simulink model "task2"  (R2024a)
settings: Solver=VariableStepAuto  StartTime=0.0  StopTime=10.0  MaxStep=0.01  RelTol=1e-3
undefined symbols (not defined in the file): Ab, Bb, Cb, D, Kb, L, xf0, xf0_hat
settings Model: Creator=sizgr  LastModifiedBy=sizgr

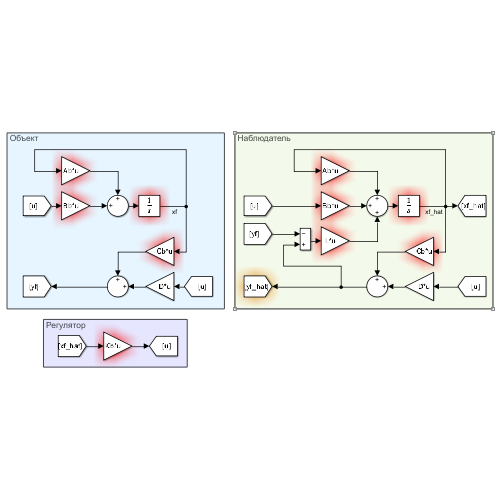
[thumbnail: Simulink's stored preview of the top-level diagram]
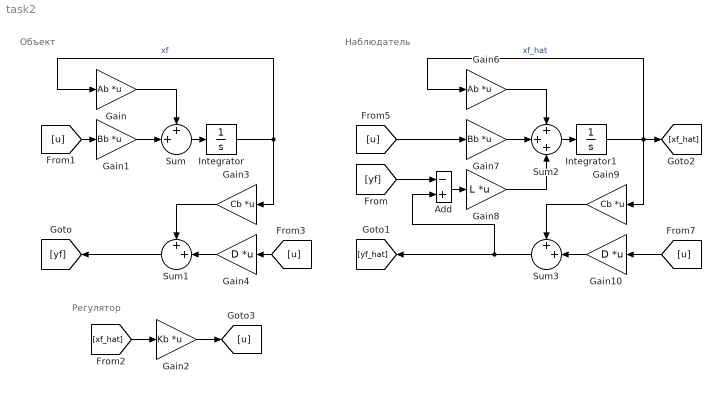
== system task2 ==
  note: Регулятор
  note: Объект
  note: Наблюдатель
  Add : Sum  Inputs=-+
  Gain : Gain  Gain=Ab  Multiplication=Matrix(K*u)
  Gain1 : Gain  Gain=Bb  Multiplication=Matrix(K*u)
  Gain10 : Gain  Gain=D  Multiplication=Matrix(K*u)
  Gain2 : Gain  Gain=Kb  Multiplication=Matrix(K*u)
  Gain3 : Gain  Gain=Cb  Multiplication=Matrix(K*u)
  Gain4 : Gain  Gain=D  Multiplication=Matrix(K*u)
  Gain6 : Gain  Gain=Ab  Multiplication=Matrix(K*u)
  Gain7 : Gain  Gain=Bb  Multiplication=Matrix(K*u)
  Gain8 : Gain  Gain=L  Multiplication=Matrix(K*u)
  Gain9 : Gain  Gain=Cb  Multiplication=Matrix(K*u)
  Integrator : Integrator  InitialCondition=xf0
  Integrator1 : Integrator  InitialCondition=xf0_hat
  Sum : Sum  Inputs=++|
  Sum1 : Sum  Inputs=++|
  Sum2 : Sum  Inputs=+++
  Sum3 : Sum  Inputs=++|
  wires:
  Sum/1 -> Integrator/1
  Integrator/1 -> Gain/1, Gain3/1  "xf"
  [u] -> Gain1/1
  Gain/1 -> Sum/1
  Gain1/1 -> Sum/2
  Gain4/1 -> Sum1/2
  [u] -> Gain4/1
  Gain3/1 -> Sum1/1
  Sum1/1 -> [yf]
  Gain9/1 -> Sum3/1
  [u] -> Gain10/1
  Gain10/1 -> Sum3/2
  Sum2/1 -> Integrator1/1
  Integrator1/1 -> Gain9/1, [xf_hat], Gain6/1  "xf_hat"
  Gain7/1 -> Sum2/2
  Sum3/1 -> Add/2, [yf_hat]
  Gain8/1 -> Sum2/3
  Add/1 -> Gain8/1
  [u] -> Gain7/1
  Gain6/1 -> Sum2/1
  [yf] -> Add/1
  [xf_hat] -> Gain2/1
  Gain2/1 -> [u]
